simulink model "benign"  (R2017a)
settings: Solver=FixedStepDiscrete  StartTime=0.0  StopTime=100  FixedStep=1  RelTol=1e-3
model workspace (MAT data in the model file):
  MCOS : class17 (value not decoded)
undefined symbols (not defined in the file or in its folder): contractAfterSimulation, contractBeforeSimulation, saveValidatorParameters
undefined symbols (not defined in the file): ContractBlock, ContractGuaranteeBlock, ContractValidatorBlock
libraries: simulink x436, CoCoSimSpecification x31
(part 2 of 3)

== system benign/uas/autonomous_flight ==
  dest_reached : Inport  OutDataTypeStr=boolean
  payload_performed : Inport  Port=2  OutDataTypeStr=boolean
  mission1_waypoint_x : Inport  Port=3  OutDataTypeStr=int32
  mission1_waypoint_y : Inport  Port=4  OutDataTypeStr=int32
  mission1_payload : Inport  Port=5  OutDataTypeStr=int32
  mission1_status : Inport  Port=6  OutDataTypeStr=int32
  mission2_waypoint_x : Inport  Port=7  OutDataTypeStr=int32
  mission2_waypoint_y : Inport  Port=8  OutDataTypeStr=int32
  mission2_payload : Inport  Port=9  OutDataTypeStr=int32
  mission2_status : Inport  Port=10  OutDataTypeStr=int32
  mission3_waypoint_x : Inport  Port=11  OutDataTypeStr=int32
  mission3_waypoint_y : Inport  Port=12  OutDataTypeStr=int32
  mission3_payload : Inport  Port=13  OutDataTypeStr=int32
  mission3_status : Inport  Port=14  OutDataTypeStr=int32
  mstate : Inport  Port=15  OutDataTypeStr=int32
  payload : Subsystem
  upd_1_status : Subsystem
  upd_2_status : Subsystem
  upd_3_status : Subsystem
  waypoint_x : Subsystem
  waypoint_y : Subsystem
  upd_mission1_waypoint_x : Outport  OutDataTypeStr=int32
  upd_mission1_waypoint_y : Outport  Port=2  OutDataTypeStr=int32
  upd_mission1_payload : Outport  Port=3  OutDataTypeStr=int32
  upd_mission1_status : Outport  Port=4  OutDataTypeStr=int32
  upd_mission2_waypoint_x : Outport  Port=5  OutDataTypeStr=int32
  upd_mission2_waypoint_y : Outport  Port=6  OutDataTypeStr=int32
  upd_mission2_payload : Outport  Port=7  OutDataTypeStr=int32
  upd_mission2_status : Outport  Port=8  OutDataTypeStr=int32
  upd_mission3_waypoint_x : Outport  Port=9  OutDataTypeStr=int32
  upd_mission3_waypoint_y : Outport  Port=10  OutDataTypeStr=int32
  upd_mission3_payload : Outport  Port=11  OutDataTypeStr=int32
  upd_mission3_status : Outport  Port=12  OutDataTypeStr=int32
  waypointPos_x : Outport  Port=13  OutDataTypeStr=int32
  waypointPos_y : Outport  Port=14  OutDataTypeStr=int32
  payloadCMD : Outport  Port=15  OutDataTypeStr=int32
  wires:
  payload/1(payloadCMD) -> payloadCMD/1
  dest_reached/1 -> payload/1(dest_reached), upd_3_status/1(dest_reached), upd_2_status/1(dest_reached), upd_1_status/1(dest_reached), waypoint_y/1(dest_reached), waypoint_x/1(dest_reached)
  payload_performed/1 -> payload/2(payload_performed), upd_3_status/2(payload_performed), upd_2_status/2(payload_performed), upd_1_status/2(payload_performed), waypoint_y/2(payload_performed), waypoint_x/2(payload_performed)
  mission1_payload/1 -> payload/3(mission1_payload), upd_mission1_payload/1
  mission1_status/1 -> payload/4(mission1_status), upd_3_status/3(mission1_status), upd_2_status/3(mission1_status), upd_1_status/3(mission1_status), waypoint_y/3(mission1_status), waypoint_x/3(mission1_status)
  mission2_payload/1 -> payload/5(mission2_payload), upd_mission2_payload/1
  mission2_status/1 -> payload/6(mission2_status), upd_3_status/4(mission2_status), upd_2_status/4(mission2_status), upd_1_status/4(mission2_status), waypoint_y/4(mission2_status), waypoint_x/4(mission2_status)
  mission3_payload/1 -> payload/7(mission3_payload), upd_mission3_payload/1
  mission3_status/1 -> payload/8(mission3_status), upd_3_status/5(mission3_status), upd_2_status/5(mission3_status), upd_1_status/5(mission3_status), waypoint_y/5(mission3_status), waypoint_x/5(mission3_status)
  mstate/1 -> payload/9(mstate), upd_3_status/6(mstate), upd_2_status/6(mstate), upd_1_status/6(mstate), waypoint_y/6(mstate), waypoint_x/6(mstate)
  waypoint_x/1(waypointPos_x) -> waypointPos_x/1
  mission1_waypoint_x/1 -> upd_mission1_waypoint_x/1, waypoint_x/7(mission1_waypoint_x)
  mission2_waypoint_x/1 -> upd_mission2_waypoint_x/1, waypoint_x/8(mission2_waypoint_x)
  mission3_waypoint_x/1 -> upd_mission3_waypoint_x/1, waypoint_x/9(mission3_waypoint_x)
  mission1_waypoint_y/1 -> upd_mission1_waypoint_y/1, waypoint_y/7(mission1_waypoint_y)
  mission2_waypoint_y/1 -> upd_mission2_waypoint_y/1, waypoint_y/8(mission2_waypoint_y)
  mission3_waypoint_y/1 -> upd_mission3_waypoint_y/1, waypoint_y/9(mission3_waypoint_y)
  waypoint_y/1(waypointPos_y) -> waypointPos_y/1
  upd_1_status/1(upd_mission1_status) -> upd_mission1_status/1
  upd_2_status/1(upd_mission2_status) -> upd_mission2_status/1
  upd_3_status/1(upd_mission3_status) -> upd_mission3_status/1

== system benign/uas/battery_health_check ==
  battery_level : Inport  OutDataTypeStr=int32
  Constant : Constant  OutDataTypeStr=int32
  Constant1 : Constant  Value=0  OutDataTypeStr=int32
  Constant2 : Constant  Value=-1  OutDataTypeStr=int32
  Logical Operator : Logic  IconShape=distinctive  AllPortsSameDT=off  OutDataTypeStr=boolean
  Relational Operator : RelationalOperator  Operator=>  OutDataTypeStr=boolean  RndMeth=Simplest
  Relational Operator1 : RelationalOperator  Operator=<=  OutDataTypeStr=boolean  RndMeth=Simplest
  Relational Operator2 : RelationalOperator  OutDataTypeStr=boolean  RndMeth=Simplest
  Switch : Switch  Criteria=u2 > Threshold
  Switch1 : Switch  Criteria=u2 > Threshold
  first_level : Constant  Value=10  OutDataTypeStr=int32
  second_level : Constant  Value=5  OutDataTypeStr=int32
  ATE7 : Outport  OutDataTypeStr=int32
  wires:
  battery_level/1 -> Relational Operator2/1, Relational Operator1/1, Relational Operator/1
  first_level/1 -> Relational Operator1/2, Relational Operator/2
  Switch/1 -> ATE7/1
  Relational Operator/1 -> Switch/2
  Constant/1 -> Switch/1
  Switch1/1 -> Switch/3
  Relational Operator1/1 -> Logical Operator/1
  Relational Operator2/1 -> Logical Operator/2
  second_level/1 -> Relational Operator2/2
  Logical Operator/1 -> Switch1/2
  Constant1/1 -> Switch1/1
  Constant2/1 -> Switch1/3

== system benign/uas/channel_afl2act ==
  in_payloadCMD : Inport  OutDataTypeStr=int32
  out_payloadCMD : Outport  OutDataTypeStr=int32
  wires:
  in_payloadCMD/1 -> out_payloadCMD/1

== system benign/uas/channel_gps2pes ==
  currPos_x : Inport  OutDataTypeStr=int32
  currPos_y : Inport  Port=2  OutDataTypeStr=int32
  currDir : Inport  Port=3  OutDataTypeStr=int32
  gps2pes_GPS_pos_x : Outport  OutDataTypeStr=int32
  gps2pes_GPS_pos_y : Outport  Port=2  OutDataTypeStr=int32
  gps2pes_GPS_dir : Outport  Port=3  OutDataTypeStr=int32
  wires:
  currPos_x/1 -> gps2pes_GPS_pos_x/1
  currPos_y/1 -> gps2pes_GPS_pos_y/1
  currDir/1 -> gps2pes_GPS_dir/1

== system benign/uas/channel_poe2mix_a ==
  in_dir : Inport  OutDataTypeStr=int32
  out_dir : Outport  OutDataTypeStr=int32
  wires:
  in_dir/1 -> out_dir/1

== system benign/uas/channel_poe2mix_b ==
  in_movement : Inport  OutDataTypeStr=int32
  out_movement : Outport  OutDataTypeStr=int32
  wires:
  in_movement/1 -> out_movement/1

== system benign/uas/done logic ==
  mission1_status : Inport  OutDataTypeStr=int32
  mission2_status : Inport  Port=2  OutDataTypeStr=int32
  mission3_status : Inport  Port=3  OutDataTypeStr=int32
  Compare To Constant : simulink/Logic and Bit Operations/Compare To Constant  relop===  const=0  OutDataTypeStr=boolean
  Compare To Constant1 : simulink/Logic and Bit Operations/Compare To Constant  relop===  const=0  OutDataTypeStr=boolean
  Compare To Constant2 : simulink/Logic and Bit Operations/Compare To Constant  relop===  const=0  OutDataTypeStr=boolean
  Compare To Constant3 : simulink/Logic and Bit Operations/Compare To Constant  relop===  const=1  OutDataTypeStr=boolean
  Compare To Constant4 : simulink/Logic and Bit Operations/Compare To Constant  relop===  const=1  OutDataTypeStr=boolean
  Compare To Constant5 : simulink/Logic and Bit Operations/Compare To Constant  relop===  const=1  OutDataTypeStr=boolean
  Logical Operator : Logic  Inputs=3  IconShape=distinctive  AllPortsSameDT=off  OutDataTypeStr=boolean
  Logical Operator1 : Logic  Inputs=3  IconShape=distinctive  AllPortsSameDT=off  OutDataTypeStr=boolean
  Switch : Switch  Criteria=u2 > Threshold
  Switch1 : Switch  Criteria=u2 > Threshold
  false : Constant  Value=0  OutDataTypeStr=boolean
  true : Constant  OutDataTypeStr=boolean
  true1 : Constant  OutDataTypeStr=boolean
  done : Outport  OutDataTypeStr=boolean
  wires:
  mission1_status/1 -> Compare To Constant/1, Compare To Constant3/1
  true/1 -> Switch/1
  Switch/1 -> done/1
  Logical Operator/1 -> Switch/2
  Compare To Constant/1 -> Logical Operator/1
  Compare To Constant1/1 -> Logical Operator/2
  mission2_status/1 -> Compare To Constant4/1, Compare To Constant1/1
  mission3_status/1 -> Compare To Constant5/1, Compare To Constant2/1
  Compare To Constant2/1 -> Logical Operator/3
  Compare To Constant3/1 -> Logical Operator1/1
  Compare To Constant4/1 -> Logical Operator1/2
  Compare To Constant5/1 -> Logical Operator1/3
  Logical Operator1/1 -> Switch1/2
  true1/1 -> Switch1/1
  false/1 -> Switch1/3
  Switch1/1 -> Switch/3

== system benign/uas/mission_planner ==
  dummy : Inport  OutDataTypeStr=boolean
  c{,1,3,7} (4 alike) : Constant  OutDataTypeStr=int32
  c10 : Constant  Value=3  OutDataTypeStr=int32
  c11 : Constant  Value=3  OutDataTypeStr=int32
  c{2,4..5,8} (4 alike) : Constant  Value=2  OutDataTypeStr=int32
  c6 : Constant  Value=0  OutDataTypeStr=int32
  c9 : Constant  Value=3  OutDataTypeStr=int32
  m1_waypoint_x : Outport  OutDataTypeStr=int32
  m1_waypoint_y : Outport  Port=2  OutDataTypeStr=int32
  m1_payload : Outport  Port=3  OutDataTypeStr=int32
  m1_status : Outport  Port=4  OutDataTypeStr=int32
  m2_waypoint_x : Outport  Port=5  OutDataTypeStr=int32
  m2_waypoint_y : Outport  Port=6  OutDataTypeStr=int32
  m2_payload : Outport  Port=7  OutDataTypeStr=int32
  m2_status : Outport  Port=8  OutDataTypeStr=int32
  m3_waypoint_x : Outport  Port=9  OutDataTypeStr=int32
  m3_waypoint_y : Outport  Port=10  OutDataTypeStr=int32
  m3_payload : Outport  Port=11  OutDataTypeStr=int32
  m3_status : Outport  Port=12  OutDataTypeStr=int32
  wires:
  c/1 -> m1_waypoint_x/1
  c1/1 -> m2_waypoint_x/1
  c2/1 -> m3_waypoint_x/1
  c3/1 -> m1_waypoint_y/1
  c4/1 -> m2_waypoint_y/1
  c5/1 -> m3_waypoint_y/1
  c6/1 -> m1_payload/1
  c7/1 -> m2_payload/1
  c8/1 -> m3_payload/1
  c9/1 -> m1_status/1
  c11/1 -> m3_status/1
  c10/1 -> m2_status/1

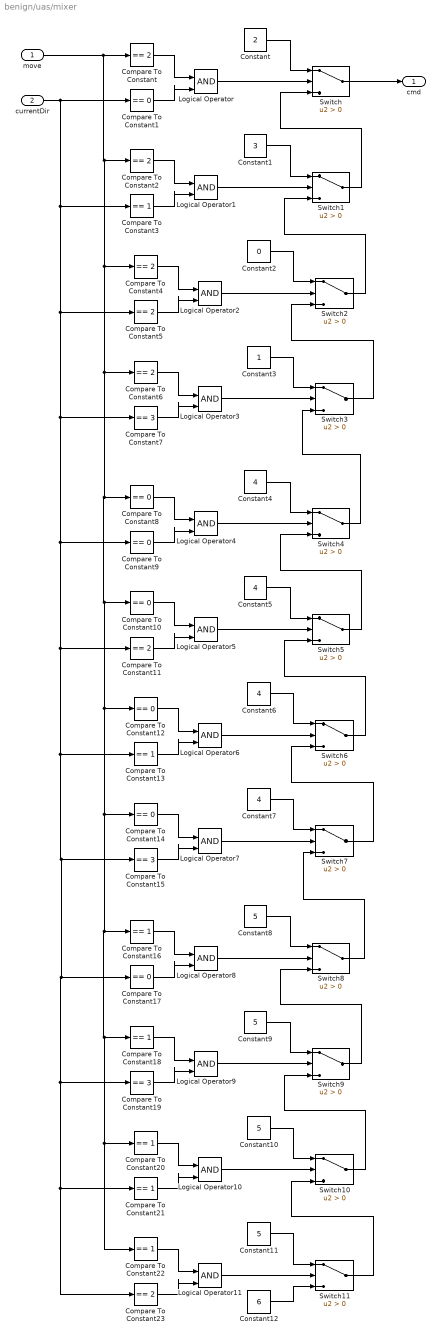
== system benign/uas/mixer ==
  move : Inport  OutDataTypeStr=int32
  currentDir : Inport  Port=2  OutDataTypeStr=int32
  Compare To Constant{,2,4..6,11,23} (7 alike) : simulink/Logic and Bit Operations/Compare To Constant  relop===  const=2  OutDataTypeStr=boolean
  Compare To Constant{1,8..10,12,14,17} (7 alike) : simulink/Logic and Bit Operations/Compare To Constant  relop===  const=0  OutDataTypeStr=boolean
  Compare To Constant{3,13,16,18,20..22} (7 alike) : simulink/Logic and Bit Operations/Compare To Constant  relop===  const=1  OutDataTypeStr=boolean
  Compare To Constant15 : simulink/Logic and Bit Operations/Compare To Constant  relop===  const=3  OutDataTypeStr=boolean
  Compare To Constant19 : simulink/Logic and Bit Operations/Compare To Constant  relop===  const=3  OutDataTypeStr=boolean
  Compare To Constant7 : simulink/Logic and Bit Operations/Compare To Constant  relop===  const=3  OutDataTypeStr=boolean
  Constant : Constant  Value=2  OutDataTypeStr=int32
  Constant1 : Constant  Value=3  OutDataTypeStr=int32
  Constant{8..11} (4 alike) : Constant  Value=5  OutDataTypeStr=int32
  Constant12 : Constant  Value=6  OutDataTypeStr=int32
  Constant2 : Constant  Value=0  OutDataTypeStr=int32
  Constant3 : Constant  OutDataTypeStr=int32
  Constant{4..7} (4 alike) : Constant  Value=4  OutDataTypeStr=int32
  Logical Operator{,1..11} (12 alike) : Logic  IconShape=distinctive  AllPortsSameDT=off  OutDataTypeStr=boolean
  Switch{,1..11} (12 alike) : Switch  Criteria=u2 > Threshold
  cmd : Outport  OutDataTypeStr=int32
  wires:
  Compare To Constant/1 -> Logical Operator/1
  Compare To Constant1/1 -> Logical Operator/2
  Logical Operator/1 -> Switch/2
  Switch/1 -> cmd/1
  Constant/1 -> Switch/1
  Logical Operator1/1 -> Switch1/2
  Compare To Constant2/1 -> Logical Operator1/1
  Switch1/1 -> Switch/3
  Compare To Constant3/1 -> Logical Operator1/2
  Constant1/1 -> Switch1/1
  Switch2/1 -> Switch1/3
  Compare To Constant4/1 -> Logical Operator2/1
  Constant2/1 -> Switch2/1
  Logical Operator2/1 -> Switch2/2
  Compare To Constant5/1 -> Logical Operator2/2
  Constant3/1 -> Switch3/1
  Switch3/1 -> Switch2/3
  Logical Operator3/1 -> Switch3/2
  Compare To Constant6/1 -> Logical Operator3/1
  Compare To Constant7/1 -> Logical Operator3/2
  Switch5/1 -> Switch4/3
  Logical Operator4/1 -> Switch4/2
  Logical Operator6/1 -> Switch6/2
  Constant6/1 -> Switch6/1
  Compare To Constant12/1 -> Logical Operator6/1
  Switch6/1 -> Switch5/3
  Switch7/1 -> Switch6/3
  Compare To Constant13/1 -> Logical Operator6/2
  Compare To Constant14/1 -> Logical Operator7/1
  Compare To Constant15/1 -> Logical Operator7/2
  Constant7/1 -> Switch7/1
  Compare To Constant8/1 -> Logical Operator4/1
  Logical Operator7/1 -> Switch7/2
  Switch4/1 -> Switch3/3
  Compare To Constant9/1 -> Logical Operator4/2
  Constant4/1 -> Switch4/1
  Constant5/1 -> Switch5/1
  Compare To Constant10/1 -> Logical Operator5/1
  Logical Operator5/1 -> Switch5/2
  Compare To Constant11/1 -> Logical Operator5/2
  Switch9/1 -> Switch8/3
  Logical Operator8/1 -> Switch8/2
  Logical Operator10/1 -> Switch10/2
  Constant10/1 -> Switch10/1
  Compare To Constant20/1 -> Logical Operator10/1
  Switch10/1 -> Switch9/3
  Switch11/1 -> Switch10/3
  Compare To Constant21/1 -> Logical Operator10/2
  Compare To Constant22/1 -> Logical Operator11/1
  Compare To Constant23/1 -> Logical Operator11/2
  Constant11/1 -> Switch11/1
  Compare To Constant16/1 -> Logical Operator8/1
  Logical Operator11/1 -> Switch11/2
  Switch8/1 -> Switch7/3
  Compare To Constant17/1 -> Logical Operator8/2
  currentDir/1 -> Compare To Constant5/1, Compare To Constant13/1, Compare To Constant21/1, Compare To Constant23/1, Compare To Constant19/1, Compare To Constant17/1, Compare To Constant15/1, Compare To Constant11/1, Compare To Constant9/1, Compare To Constant7/1, Compare To Constant3/1, Compare To Constant1/1
  Constant8/1 -> Switch8/1
  Constant9/1 -> Switch9/1
  Compare To Constant18/1 -> Logical Operator9/1
  move/1 -> Compare To Constant22/1, Compare To Constant20/1, Compare To Constant18/1, Compare To Constant16/1, Compare To Constant14/1, Compare To Constant12/1, Compare To Constant10/1, Compare To Constant8/1, Compare To Constant6/1, Compare To Constant4/1, Compare To Constant2/1, Compare To Constant/1
  Logical Operator9/1 -> Switch9/2
  Compare To Constant19/1 -> Logical Operator9/2
  Constant12/1 -> Switch11/3

== system benign/uas/navigator ==
  estimatedPos_x : Inport  OutDataTypeStr=int32
  estimatedPos_y : Inport  Port=2  OutDataTypeStr=int32
  waypointPos_x : Inport  Port=3  OutDataTypeStr=int32
  waypointPos_y : Inport  Port=4  OutDataTypeStr=int32
  Logical Operator : Logic  IconShape=distinctive  AllPortsSameDT=off  OutDataTypeStr=boolean
  Relational Operator : RelationalOperator  Operator===  OutDataTypeStr=boolean  RndMeth=Simplest
  Relational Operator1 : RelationalOperator  Operator===  OutDataTypeStr=boolean  RndMeth=Simplest
  dest_reached : Outport  OutDataTypeStr=boolean
  wires:
  estimatedPos_x/1 -> Relational Operator/1
  waypointPos_x/1 -> Relational Operator/2
  estimatedPos_y/1 -> Relational Operator1/1
  waypointPos_y/1 -> Relational Operator1/2
  Logical Operator/1 -> dest_reached/1
  Relational Operator/1 -> Logical Operator/1
  Relational Operator1/1 -> Logical Operator/2

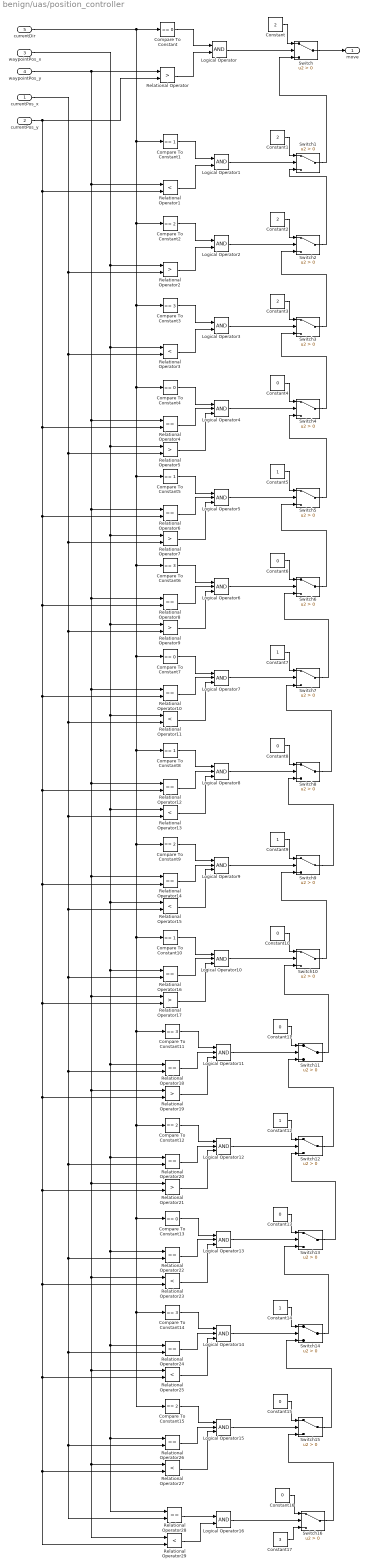
== system benign/uas/position_controller ==
  currentPos_x : Inport  OutDataTypeStr=int32
  currentPos_y : Inport  Port=2  OutDataTypeStr=int32
  waypointPos_x : Inport  Port=3  OutDataTypeStr=int32
  waypointPos_y : Inport  Port=4  OutDataTypeStr=int32
  currentDir : Inport  Port=5  OutDataTypeStr=int32
  Compare To Constant{,4,7,13} (4 alike) : simulink/Logic and Bit Operations/Compare To Constant  relop===  const=0  OutDataTypeStr=boolean
  Compare To Constant{1,5,8,10} (4 alike) : simulink/Logic and Bit Operations/Compare To Constant  relop===  const=1  OutDataTypeStr=boolean
  Compare To Constant{3,6,11,14} (4 alike) : simulink/Logic and Bit Operations/Compare To Constant  relop===  const=3  OutDataTypeStr=boolean
  Compare To Constant{2,9,12,15} (4 alike) : simulink/Logic and Bit Operations/Compare To Constant  relop===  const=2  OutDataTypeStr=boolean
  Constant{,1..3} (4 alike) : Constant  Value=2  OutDataTypeStr=int32
  Constant{4,6,8,10..11,13,15..16} (8 alike) : Constant  Value=0  OutDataTypeStr=int32
  Constant{5,7,9,12,14} (5 alike) : Constant  OutDataTypeStr=int32
  Constant17 : Constant  Value=3  OutDataTypeStr=int32
  Logical Operator{,1..3,16} (5 alike) : Logic  AllPortsSameDT=off  OutDataTypeStr=boolean
  Logical Operator{4..15} (12 alike) : Logic  Inputs=3  AllPortsSameDT=off  OutDataTypeStr=boolean
  Relational Operator{,2,5,7,9,17,19,21} (8 alike) : RelationalOperator  Operator=>  OutDataTypeStr=boolean  RndMeth=Simplest
  Relational Operator{1,3,11,13,15,23,25,27,29} (9 alike) : RelationalOperator  Operator=<  OutDataTypeStr=boolean  RndMeth=Simplest
  Relational Operator{4,6,8,10,12,14,16,18,20,22,24,26,28} (13 alike) : RelationalOperator  Operator===  OutDataTypeStr=boolean  RndMeth=Simplest
  Switch{,1..16} (17 alike) : Switch  Criteria=u2 > Threshold
  move : Outport  OutDataTypeStr=int32
  wires:
  Compare To Constant/1 -> Logical Operator/1
  Relational Operator/1 -> Logical Operator/2
  Logical Operator/1 -> Switch/2
  Switch/1 -> move/1
  Constant/1 -> Switch/1
  Constant1/1 -> Switch1/1
  Switch1/1 -> Switch/3
  Relational Operator1/1 -> Logical Operator1/2
  Logical Operator1/1 -> Switch1/2
  Compare To Constant1/1 -> Logical Operator1/1
  Switch2/1 -> Switch1/3
  Logical Operator2/1 -> Switch2/2
  Compare To Constant2/1 -> Logical Operator2/1
  Constant2/1 -> Switch2/1
  Relational Operator2/1 -> Logical Operator2/2
  Constant3/1 -> Switch3/1
  Compare To Constant3/1 -> Logical Operator3/1
  Relational Operator3/1 -> Logical Operator3/2
  Logical Operator3/1 -> Switch3/2
  Switch3/1 -> Switch2/3
  Relational Operator4/1 -> Logical Operator4/2
  Compare To Constant4/1 -> Logical Operator4/1
  Constant4/1 -> Switch4/1
  Logical Operator4/1 -> Switch4/2
  Switch4/1 -> Switch3/3
  Relational Operator5/1 -> Logical Operator4/3
  Constant5/1 -> Switch5/1
  Compare To Constant5/1 -> Logical Operator5/1
  Logical Operator5/1 -> Switch5/2
  Relational Operator7/1 -> Logical Operator5/3
  Relational Operator6/1 -> Logical Operator5/2
  Switch5/1 -> Switch4/3
  Switch6/1 -> Switch5/3
  Relational Operator8/1 -> Logical Operator6/2
  Constant6/1 -> Switch6/1
  Relational Operator9/1 -> Logical Operator6/3
  Compare To Constant6/1 -> Logical Operator6/1
  Logical Operator6/1 -> Switch6/2
  Logical Operator7/1 -> Switch7/2
  Compare To Constant7/1 -> Logical Operator7/1
  Relational Operator11/1 -> Logical Operator7/3
  Constant7/1 -> Switch7/1
  Relational Operator10/1 -> Logical Operator7/2
  Switch7/1 -> Switch6/3
  Compare To Constant8/1 -> Logical Operator8/1
  Logical Operator8/1 -> Switch8/2
  Relational Operator12/1 -> Logical Operator8/2
  Switch8/1 -> Switch7/3
  Constant8/1 -> Switch8/1
  Relational Operator13/1 -> Logical Operator8/3
  Switch9/1 -> Switch8/3
  Constant9/1 -> Switch9/1
  Relational Operator14/1 -> Logical Operator9/2
  Compare To Constant9/1 -> Logical Operator9/1
  Logical Operator9/1 -> Switch9/2
  Relational Operator15/1 -> Logical Operator9/3
  Relational Operator17/1 -> Logical Operator10/3
  Compare To Constant10/1 -> Logical Operator10/1
  Constant10/1 -> Switch10/1
  Logical Operator10/1 -> Switch10/2
  Switch10/1 -> Switch9/3
  Relational Operator16/1 -> Logical Operator10/2
  Logical Operator11/1 -> Switch11/2
  Constant11/1 -> Switch11/1
  Compare To Constant11/1 -> Logical Operator11/1
  Relational Operator19/1 -> Logical Operator11/3
  Switch11/1 -> Switch10/3
  Relational Operator18/1 -> Logical Operator11/2
  Switch12/1 -> Switch11/3
  Relational Operator20/1 -> Logical Operator12/2
  Compare To Constant12/1 -> Logical Operator12/1
  Constant12/1 -> Switch12/1
  Relational Operator21/1 -> Logical Operator12/3
  Logical Operator12/1 -> Switch12/2
  Relational Operator23/1 -> Logical Operator13/3
  Compare To Constant13/1 -> Logical Operator13/1
  Relational Operator22/1 -> Logical Operator13/2
  Constant13/1 -> Switch13/1
  Logical Operator13/1 -> Switch13/2
  Switch13/1 -> Switch12/3
  Relational Operator24/1 -> Logical Operator14/2
  Switch14/1 -> Switch13/3
  Logical Operator14/1 -> Switch14/2
  Constant14/1 -> Switch14/1
  Compare To Constant14/1 -> Logical Operator14/1
  Relational Operator25/1 -> Logical Operator14/3
  Relational Operator27/1 -> Logical Operator15/3
  Relational Operator26/1 -> Logical Operator15/2
  Logical Operator15/1 -> Switch15/2
  Constant15/1 -> Switch15/1
  Compare To Constant15/1 -> Logical Operator15/1
  Switch15/1 -> Switch14/3
  currentDir/1 -> Compare To Constant5/1, Compare To Constant6/1, Compare To Constant7/1, Compare To Constant8/1, Compare To Constant9/1, Compare To Constant10/1, Compare To Constant12/1, Compare To Constant13/1, Compare To Constant14/1, Compare To Constant15/1, Compare To Constant11/1, Compare To Constant4/1, Compare To Constant3/1, Compare To Constant2/1, Compare To Constant1/1, Compare To Constant/1
  waypointPos_x/1 -> Relational Operator5/1, Relational Operator7/1, Relational Operator9/1, Relational Operator11/1, Relational Operator13/1, Relational Operator15/1, Relational Operator16/1, Relational Operator20/1, Relational Operator22/1, Relational Operator24/1, Relational Operator26/1, Relational Operator28/1, Relational Operator18/1, Relational Operator3/1, Relational Operator2/1
  currentPos_y/1 -> Relational Operator6/2, Relational Operator8/2, Relational Operator10/2, Relational Operator12/2, Relational Operator14/2, Relational Operator17/2, Relational Operator21/2, Relational Operator23/2, Relational Operator25/2, Relational Operator27/2, Relational Operator29/2, Relational Operator19/2, Relational Operator4/2, Relational Operator1/2, Relational Operator/2
  Constant16/1 -> Switch16/1
  Relational Operator28/1 -> Logical Operator16/1
  Logical Operator16/1 -> Switch16/2
  waypointPos_y/1 -> Relational Operator/1, Relational Operator4/1, Relational Operator6/1, Relational Operator8/1, Relational Operator10/1, Relational Operator12/1, Relational Operator14/1, Relational Operator17/1, Relational Operator21/1, Relational Operator23/1, Relational Operator25/1, Relational Operator27/1, Relational Operator29/1, Relational Operator19/1, Relational Operator1/1
  Switch16/1 -> Switch15/3
  currentPos_x/1 -> Relational Operator7/2, Relational Operator9/2, Relational Operator11/2, Relational Operator13/2, Relational Operator15/2, Relational Operator16/2, Relational Operator20/2, Relational Operator22/2, Relational Operator24/2, Relational Operator26/2, Relational Operator28/2, Relational Operator18/2, Relational Operator5/2, Relational Operator3/2, Relational Operator2/2
  Relational Operator29/1 -> Logical Operator16/2
  Constant17/1 -> Switch16/3

== system benign/uas/position_estimator ==
  gps2pes_GPS_pos_x : Inport  OutDataTypeStr=int32
  gps2pes_GPS_pos_y : Inport  Port=2  OutDataTypeStr=int32
  gps2pes_GPS_dir : Inport  Port=3  OutDataTypeStr=int32
  currPos_x : Inport  Port=4  OutDataTypeStr=int32
  currPos_y : Inport  Port=5  OutDataTypeStr=int32
  currDir : Inport  Port=6  OutDataTypeStr=int32
  estimatedPos_x : Outport  OutDataTypeStr=int32
  estimatedPos_y : Outport  Port=2  OutDataTypeStr=int32
  estimatedDir : Outport  Port=3  OutDataTypeStr=int32
  wires:
  gps2pes_GPS_pos_x/1 -> estimatedPos_x/1
  gps2pes_GPS_pos_y/1 -> estimatedPos_y/1
  gps2pes_GPS_dir/1 -> estimatedDir/1

== system benign/uas/state_machine ==
  ATE6 : Inport
  ATE7 : Inport  Port=2
  six : Constant  Value=6  OutDataTypeStr=int32
  mstate : Outport  OutDataTypeStr=int32
  wires:
  six/1 -> mstate/1

== system benign/uas/yaw2dir ==
  yaw : Inport  OutDataTypeStr=int32
  Switch : Switch  Criteria=u2 > Threshold
  Switch1 : Switch  Criteria=u2 > Threshold
  Switch2 : Switch  Criteria=u2 > Threshold
  c0 : Constant  Value=0  OutDataTypeStr=int32
  c1 : Constant  OutDataTypeStr=int32
  c2 : Constant  Value=2  OutDataTypeStr=int32
  c3 : Constant  Value=3  OutDataTypeStr=int32
  yaw == 0 : simulink/Logic and Bit Operations/Compare To Constant  relop===  const=0  OutDataTypeStr=boolean
  yaw == 1 : simulink/Logic and Bit Operations/Compare To Constant  relop===  const=1  OutDataTypeStr=boolean
  yaw == 2 : simulink/Logic and Bit Operations/Compare To Constant  relop===  const=2  OutDataTypeStr=boolean
  dir : Outport  OutDataTypeStr=int32
  wires:
  yaw/1 -> yaw == 2/1, yaw == 1/1, yaw == 0/1
  yaw == 0/1 -> Switch/2
  c0/1 -> Switch/1
  Switch/1 -> dir/1
  yaw == 1/1 -> Switch1/2
  c2/1 -> Switch1/1
  Switch1/1 -> Switch/3
  yaw == 2/1 -> Switch2/2
  c1/1 -> Switch2/1
  c3/1 -> Switch2/3
  Switch2/1 -> Switch1/3

== system benign/uas/RC_receiver_health_check/duration ==
  p : Inport  OutDataTypeStr=boolean
  Add : Sum
  Constant : Constant  OutDataTypeStr=int32
  Constant1 : Constant  Value=0  OutDataTypeStr=int32
  Constant2 : Constant  Value=0  OutDataTypeStr=int32
  Constant3 : Constant  OutDataTypeStr=int32
  Logical Operator : Logic  Operator=NOT  IconShape=distinctive  AllPortsSameDT=off  OutDataTypeStr=boolean
  Switch : Switch  Criteria=u2 > Threshold
  Switch1 : Switch  Criteria=u2 > Threshold
  Unit Delay : UnitDelay  SampleTime=-1
  arrow1 : CoCoSimSpecification/arrow  LustreOperatorBlock=ArrowOperator
      settings: SourceProductName=CoCoSim Specification
  r : Outport  OutDataTypeStr=int32
  wires:
  Switch/1 -> arrow1/1
  arrow1/1 -> Unit Delay/1, r/1
  p/1 -> Logical Operator/1
  Logical Operator/1 -> Switch1/2, Switch/2
  Switch1/1 -> arrow1/2
  Constant/1 -> Switch/1
  Constant1/1 -> Switch/3
  Constant2/1 -> Switch1/3
  Constant3/1 -> Add/1
  Unit Delay/1 -> Add/2
  Add/1 -> Switch1/1

== system benign/uas/actuator/Subsystem ==
  cmd : Inport  OutDataTypeStr=int32
  Compare To Constant : simulink/Logic and Bit Operations/Compare To Constant  relop===  const=2  OutDataTypeStr=boolean
  Compare To Constant1 : simulink/Logic and Bit Operations/Compare To Constant  relop===  const=0  OutDataTypeStr=boolean
  Compare To Constant2 : simulink/Logic and Bit Operations/Compare To Constant  relop===  const=3  OutDataTypeStr=boolean
  Compare To Constant3 : simulink/Logic and Bit Operations/Compare To Constant  relop===  const=1  OutDataTypeStr=boolean
  Compare To Constant4 : simulink/Logic and Bit Operations/Compare To Constant  relop===  const=6  OutDataTypeStr=boolean
  Switch{,1..4} (5 alike) : Switch  Criteria=u2 > Threshold
  false : Constant  OutDataTypeStr=boolean
  true{,1..4} (5 alike) : Constant  OutDataTypeStr=boolean
  battery4pos_consumed : Outport
  wires:
  Switch/1 -> battery4pos_consumed/1
  true/1 -> Switch/1
  Compare To Constant/1 -> Switch/2
  Switch1/1 -> Switch/3
  Switch2/1 -> Switch1/3
  Switch3/1 -> Switch2/3
  true1/1 -> Switch1/1
  Compare To Constant1/1 -> Switch1/2
  true2/1 -> Switch2/1
  Compare To Constant2/1 -> Switch2/2
  true3/1 -> Switch3/1
  Compare To Constant3/1 -> Switch3/2
  Switch4/1 -> Switch3/3
  Compare To Constant4/1 -> Switch4/2
  true4/1 -> Switch4/1
  cmd/1 -> Compare To Constant2/1, Compare To Constant4/1, Compare To Constant3/1, Compare To Constant1/1, Compare To Constant/1
  false/1 -> Switch4/3

== system benign/uas/actuator/Subsystem1 ==
  cmd : Inport  OutDataTypeStr=int32
  currentPos_x : Inport  Port=2  OutDataTypeStr=int32
  Add : Sum
  Add1 : Sum
  Compare To Constant : simulink/Logic and Bit Operations/Compare To Constant  relop===  const=2  OutDataTypeStr=boolean
  Compare To Constant1 : simulink/Logic and Bit Operations/Compare To Constant  relop===  const=0  OutDataTypeStr=boolean
  Compare To Constant2 : simulink/Logic and Bit Operations/Compare To Constant  relop===  const=3  OutDataTypeStr=boolean
  Compare To Constant3 : simulink/Logic and Bit Operations/Compare To Constant  relop===  const=1  OutDataTypeStr=boolean
  Compare To Constant4 : simulink/Logic and Bit Operations/Compare To Constant  relop===  const=6  OutDataTypeStr=boolean
  Constant : Constant  OutDataTypeStr=int32
  Constant1 : Constant  Value=-1  OutDataTypeStr=int32
  Switch{,1..4} (5 alike) : Switch  Criteria=u2 > Threshold
  nextPos_x : Outport
  wires:
  cmd/1 -> Compare To Constant/1, Compare To Constant1/1, Compare To Constant3/1, Compare To Constant4/1, Compare To Constant2/1
  Compare To Constant4/1 -> Switch4/2
  Switch4/1 -> Switch3/3
  Compare To Constant3/1 -> Switch3/2
  Compare To Constant2/1 -> Switch2/2
  Compare To Constant1/1 -> Switch1/2
  Switch3/1 -> Switch2/3
  Switch2/1 -> Switch1/3
  Switch1/1 -> Switch/3
  Compare To Constant/1 -> Switch/2
  Switch/1 -> nextPos_x/1
  Constant/1 -> Add/2
  Add/1 -> Switch1/1
  Add1/1 -> Switch3/1
  Constant1/1 -> Add1/2
  currentPos_x/1 -> Switch4/3, Switch4/1, Add1/1, Switch2/1, Add/1, Switch/1

== system benign/uas/actuator/Subsystem2 ==
  cmd : Inport  OutDataTypeStr=int32
  currentPos_y : Inport  Port=2  OutDataTypeStr=int32
  Add2 : Sum
  Add3 : Sum
  Compare To Constant : simulink/Logic and Bit Operations/Compare To Constant  relop===  const=2  OutDataTypeStr=boolean
  Compare To Constant1 : simulink/Logic and Bit Operations/Compare To Constant  relop===  const=0  OutDataTypeStr=boolean
  Compare To Constant2 : simulink/Logic and Bit Operations/Compare To Constant  relop===  const=3  OutDataTypeStr=boolean
  Compare To Constant3 : simulink/Logic and Bit Operations/Compare To Constant  relop===  const=1  OutDataTypeStr=boolean
  Compare To Constant4 : simulink/Logic and Bit Operations/Compare To Constant  relop===  const=6  OutDataTypeStr=boolean
  Constant2 : Constant  OutDataTypeStr=int32
  Constant3 : Constant  Value=-1  OutDataTypeStr=int32
  Switch{,1..4} (5 alike) : Switch  Criteria=u2 > Threshold
  nextPos_y : Outport
  wires:
  currentPos_y/1 -> Add2/1, Switch1/1, Add3/1, Switch4/1, Switch4/3, Switch3/1
  Switch/1 -> nextPos_y/1
  Compare To Constant/1 -> Switch/2
  Switch1/1 -> Switch/3
  Switch2/1 -> Switch1/3
  Switch3/1 -> Switch2/3
  Compare To Constant1/1 -> Switch1/2
  Compare To Constant2/1 -> Switch2/2
  Compare To Constant3/1 -> Switch3/2
  Switch4/1 -> Switch3/3
  Compare To Constant4/1 -> Switch4/2
  cmd/1 -> Compare To Constant2/1, Compare To Constant4/1, Compare To Constant3/1, Compare To Constant1/1, Compare To Constant/1
  Constant2/1 -> Add2/2
  Add2/1 -> Switch/1
  Constant3/1 -> Add3/2
  Add3/1 -> Switch2/1

== system benign/uas/actuator/choose_battery_consumption ==
  i : Inport  OutDataTypeStr=int32
  one : Constant  OutDataTypeStr=int32
  o : Outport  OutDataTypeStr=int32
  wires:
  one/1 -> o/1

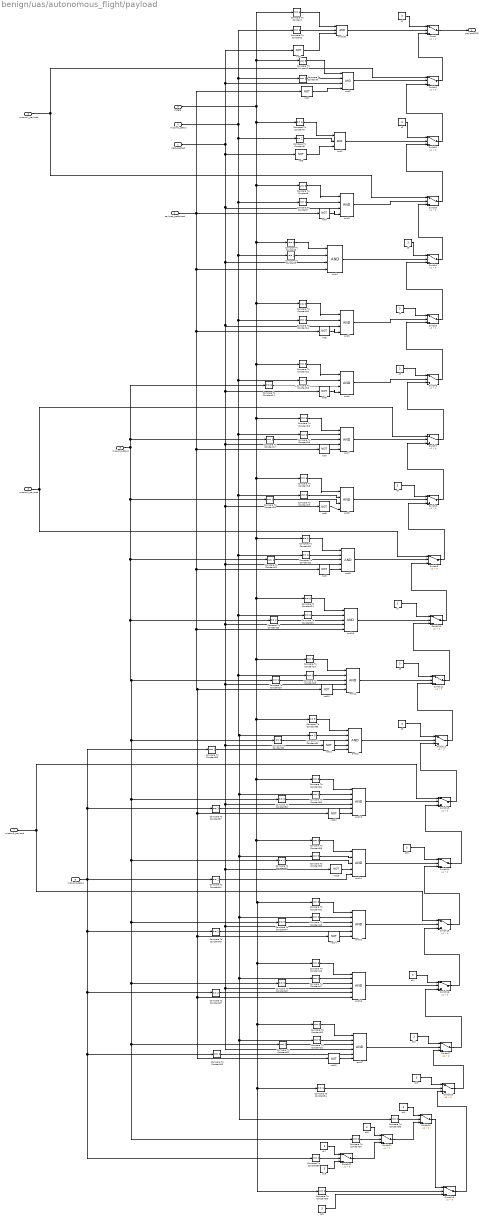
== system benign/uas/autonomous_flight/payload ==
  dest_reached : Inport  OutDataTypeStr=boolean
  payload_performed : Inport  Port=2  OutDataTypeStr=boolean
  mission1_payload : Inport  Port=3  OutDataTypeStr=int32
  mission1_status : Inport  Port=4  OutDataTypeStr=int32
  mission2_payload : Inport  Port=5  OutDataTypeStr=int32
  mission2_status : Inport  Port=6  OutDataTypeStr=int32
  mission3_payload : Inport  Port=7  OutDataTypeStr=int32
  mission3_status : Inport  Port=8  OutDataTypeStr=int32
  mstate : Inport  Port=9  OutDataTypeStr=int32
  Compare To Constant{,2,4,6,8,10,12,15,18,21,24,27,30,34,38,42,46,50} (18 alike) : simulink/Logic and Bit Operations/Compare To Constant  relop===  const=6  OutDataTypeStr=boolean
  Compare To Constant{1,3,14,17,33,37,54} (7 alike) : simulink/Logic and Bit Operations/Compare To Constant  relop===  const=3  OutDataTypeStr=boolean
  Compare To Constant{5,7,9,11,20,23,26,29,41,45,49,53,56..58} (15 alike) : simulink/Logic and Bit Operations/Compare To Constant  relop===  const=2  OutDataTypeStr=boolean
  Compare To Constant{13,16,19,22,25,28,31..32,35..36,39..40,43..44,47..48,51..52} (18 alike) : simulink/Logic and Bit Operations/Compare To Constant  relop===  const=0  OutDataTypeStr=boolean
  Compare To Constant55 : simulink/Logic and Bit Operations/Compare To Constant  relop===  const=4  OutDataTypeStr=boolean
  Switch{,1..22} (23 alike) : Switch  Criteria=u2 > Threshold
  and1 : Logic  Inputs=3  IconShape=distinctive  AllPortsSameDT=off  OutDataTypeStr=boolean
  and{7,9..12,14} (6 alike) : Logic  Inputs=5  IconShape=distinctive  AllPortsSameDT=off  OutDataTypeStr=boolean
  and101 : Logic  Inputs=3  IconShape=distinctive  AllPortsSameDT=off  OutDataTypeStr=boolean
  and{13,15..17} (4 alike) : Logic  Inputs=6  IconShape=distinctive  AllPortsSameDT=off  OutDataTypeStr=boolean
  and{2..6,8} (6 alike) : Logic  Inputs=4  IconShape=distinctive  AllPortsSameDT=off  OutDataTypeStr=boolean
  c{1..18} (18 alike) : Constant  Value=3  OutDataTypeStr=int32
  not{1..15} (15 alike) : Logic  Operator=NOT  Inputs=3  IconShape=distinctive  AllPortsSameDT=off  OutDataTypeStr=boolean
  payloadCMD : Outport  OutDataTypeStr=int32
  wires:
  Switch/1 -> payloadCMD/1
  c1/1 -> Switch/1
  and101/1 -> Switch/2
  Compare To Constant/1 -> and101/1
  Compare To Constant1/1 -> and101/2
  not1/1 -> and101/3
  Compare To Constant3/1 -> and2/2
  Compare To Constant2/1 -> and2/1
  Switch1/1 -> Switch/3
  and2/1 -> Switch1/2
  not2/1 -> and2/4
  Switch2/1 -> Switch1/3
  Compare To Constant4/1 -> and1/1
  c2/1 -> Switch2/1
  Compare To Constant5/1 -> and1/2
  and1/1 -> Switch2/2
  not3/1 -> and1/3
  and3/1 -> Switch3/2
  Compare To Constant7/1 -> and3/2
  Switch3/1 -> Switch2/3
  Compare To Constant6/1 -> and3/1
  not4/1 -> and3/4
  Compare To Constant8/1 -> and4/1
  and4/1 -> Switch4/2
  Compare To Constant9/1 -> and4/2
  Switch4/1 -> Switch3/3
  c3/1 -> Switch4/1
  Compare To Constant10/1 -> and5/1
  Compare To Constant11/1 -> and5/2
  and5/1 -> Switch5/2
  mission1_payload/1 -> Switch3/1, Switch1/1
  not5/1 -> and5/4
  Switch5/1 -> Switch4/3
  c4/1 -> Switch5/1
  Compare To Constant13/1 -> and6/2
  Compare To Constant12/1 -> and6/1
  not6/1 -> and6/4
  Switch6/1 -> Switch5/3
  c5/1 -> Switch6/1
  and6/1 -> Switch6/2
  Compare To Constant14/1 -> and6/3
  Compare To Constant17/1 -> and7/3
  and7/1 -> Switch7/2
  Compare To Constant16/1 -> and7/2
  Compare To Constant15/1 -> and7/1
  Switch7/1 -> Switch6/3
  not7/1 -> and7/5
  mission2_payload/1 -> Switch9/1, Switch7/1
  Compare To Constant18/1 -> and8/1
  Compare To Constant20/1 -> and8/3
  and8/1 -> Switch8/2
  Switch8/1 -> Switch7/3
  Compare To Constant19/1 -> and8/2
  not8/1 -> and8/4
  c6/1 -> Switch8/1
  Switch9/1 -> Switch8/3
  Compare To Constant21/1 -> and9/1
  Compare To Constant23/1 -> and9/3
  and9/1 -> Switch9/2
  Compare To Constant22/1 -> and9/2
  not9/1 -> and9/5
  Switch10/1 -> Switch9/3
  and10/1 -> Switch10/2
  Compare To Constant24/1 -> and10/1
  Compare To Constant26/1 -> and10/3
  Compare To Constant25/1 -> and10/2
  c7/1 -> Switch10/1
  c8/1 -> Switch11/1
  Switch11/1 -> Switch10/3
  Compare To Constant29/1 -> and11/3
  and11/1 -> Switch11/2
  Compare To Constant28/1 -> and11/2
  Compare To Constant27/1 -> and11/1
  not10/1 -> and11/5
  c9/1 -> Switch12/1
  Compare To Constant30/1 -> and12/1
  Switch12/1 -> Switch11/3
  Compare To Constant31/1 -> and12/2
  and12/1 -> Switch12/2
  Compare To Constant32/1 -> and12/3
  not11/1 -> and12/4
  Compare To Constant33/1 -> and12/5
  Switch13/1 -> Switch12/3
  Compare To Constant37/1 -> and13/5
  and13/1 -> Switch13/2
  Compare To Constant34/1 -> and13/1
  Compare To Constant35/1 -> and13/2
  Compare To Constant36/1 -> and13/3
  not12/1 -> and13/6
  Compare To Constant40/1 -> and14/3
  Compare To Constant39/1 -> and14/2
  Compare To Constant38/1 -> and14/1
  Compare To Constant41/1 -> and14/5
  Switch14/1 -> Switch13/3
  and14/1 -> Switch14/2
  c10/1 -> Switch14/1
  not13/1 -> and14/4
  and15/1 -> Switch15/2
  Compare To Constant45/1 -> and15/5
  Compare To Constant44/1 -> and15/3
  Switch15/1 -> Switch14/3
  not14/1 -> and15/6
  Compare To Constant42/1 -> and15/1
  Compare To Constant43/1 -> and15/2
  mission3_payload/1 -> Switch13/1, Switch15/1
  Switch16/1 -> Switch15/3
  Compare To Constant46/1 -> and16/1
  and16/1 -> Switch16/2
  Compare To Constant48/1 -> and16/3
  Compare To Constant47/1 -> and16/2
  Compare To Constant49/1 -> and16/5
  c11/1 -> Switch16/1
  and17/1 -> Switch17/2
  payload_performed/1 -> not2/1, not15/1, and16/6, not14/1, not12/1, not10/1, and10/5, not9/1, not7/1, not5/1, and4/4, not4/1
  c12/1 -> Switch17/1
  Compare To Constant51/1 -> and17/2
  mission2_status/1 -> Compare To Constant14/1, Compare To Constant17/1, Compare To Constant57/1, Compare To Constant52/1, Compare To Constant48/1, Compare To Constant44/1, Compare To Constant40/1, Compare To Constant36/1, Compare To Constant32/1, Compare To Constant29/1, Compare To Constant26/1, Compare To Constant23/1, Compare To Constant20/1
  dest_reached/1 -> and2/3, not1/1, and9/4, and16/4, and17/4, and15/4, not13/1, and13/4, not11/1, and11/4, and10/4, not8/1, and7/4, not6/1, and5/3, and4/3, and3/3, not3/1
  Compare To Constant53/1 -> and17/5
  Compare To Constant50/1 -> and17/1
  mission1_status/1 -> Compare To Constant7/1, Compare To Constant56/1, Compare To Constant51/1, Compare To Constant47/1, Compare To Constant43/1, Compare To Constant39/1, Compare To Constant35/1, Compare To Constant31/1, Compare To Constant28/1, Compare To Constant25/1, Compare To Constant22/1, Compare To Constant19/1, Compare To Constant16/1, Compare To Constant13/1, Compare To Constant11/1, Compare To Constant9/1, Compare To Constant5/1, Compare To Constant3/1, Compare To Constant1/1
  Compare To Constant52/1 -> and17/3
  Switch17/1 -> Switch16/3
  not15/1 -> and17/6
  Switch18/1 -> Switch17/3
  Compare To Constant54/1 -> Switch18/2
  c13/1 -> Switch18/1
  Switch19/1 -> Switch18/3
  mstate/1 -> Compare To Constant6/1, Compare To Constant12/1, Compare To Constant27/1, Compare To Constant55/1, Compare To Constant54/1, Compare To Constant50/1, Compare To Constant46/1, Compare To Constant42/1, Compare To Constant38/1, Compare To Constant34/1, Compare To Constant30/1, Compare To Constant24/1, Compare To Constant21/1, Compare To Constant18/1, Compare To Constant15/1, Compare To Constant10/1, Compare To Constant8/1, Compare To Constant4/1, Compare To Constant2/1, Compare To Constant/1
  c15/1 -> Switch19/3
  Compare To Constant55/1 -> Switch19/2
  Compare To Constant56/1 -> Switch20/2
  c14/1 -> Switch20/1
  Switch20/1 -> Switch19/1
  c16/1 -> Switch21/1
  Compare To Constant57/1 -> Switch21/2
  Switch21/1 -> Switch20/3
  Compare To Constant58/1 -> Switch22/2
  Switch22/1 -> Switch21/3
  c17/1 -> Switch22/1
  mission3_status/1 -> Compare To Constant33/1, Compare To Constant37/1, Compare To Constant49/1, Compare To Constant58/1, Compare To Constant53/1, Compare To Constant45/1, Compare To Constant41/1
  c18/1 -> Switch22/3

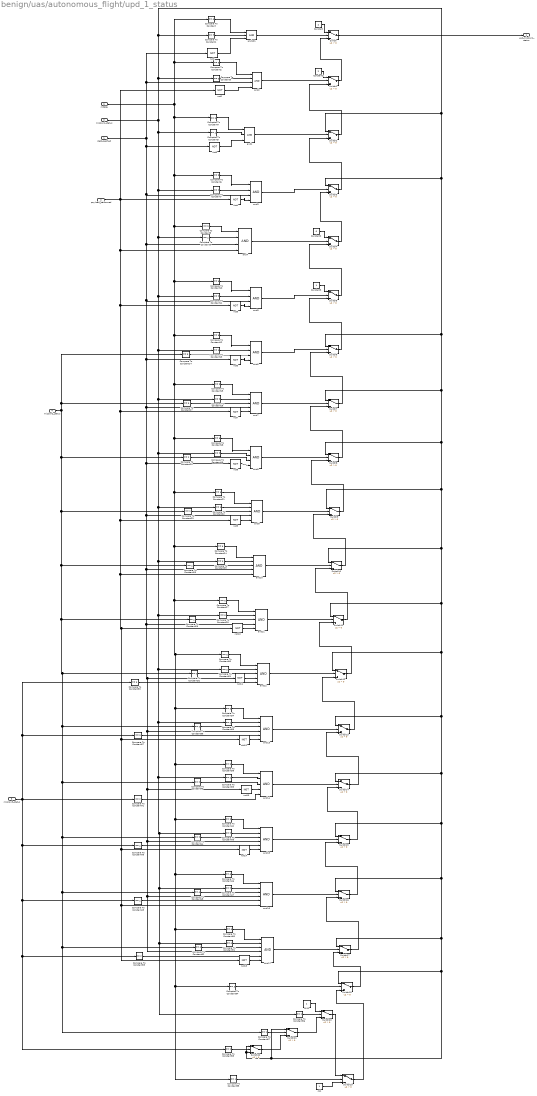
== system benign/uas/autonomous_flight/upd_1_status ==
  dest_reached : Inport  OutDataTypeStr=boolean
  payload_performed : Inport  Port=2  OutDataTypeStr=boolean
  mission1_status : Inport  Port=3  OutDataTypeStr=int32
  mission2_status : Inport  Port=4  OutDataTypeStr=int32
  mission3_status : Inport  Port=5  OutDataTypeStr=int32
  mstate : Inport  Port=6  OutDataTypeStr=int32
  Compare To Constant{,2,4,6,8,10,12,15,18,21,24,27,30,34,38,42,46,50} (18 alike) : simulink/Logic and Bit Operations/Compare To Constant  relop===  const=6  OutDataTypeStr=boolean
  Compare To Constant{1,3,14,17,33,37,54} (7 alike) : simulink/Logic and Bit Operations/Compare To Constant  relop===  const=3  OutDataTypeStr=boolean
  Compare To Constant{5,7,9,11,20,23,26,29,41,45,49,53,56..58} (15 alike) : simulink/Logic and Bit Operations/Compare To Constant  relop===  const=2  OutDataTypeStr=boolean
  Compare To Constant{13,16,19,22,25,28,31..32,35..36,39..40,43..44,47..48,51..52} (18 alike) : simulink/Logic and Bit Operations/Compare To Constant  relop===  const=0  OutDataTypeStr=boolean
  Compare To Constant55 : simulink/Logic and Bit Operations/Compare To Constant  relop===  const=4  OutDataTypeStr=boolean
  Constant : Constant  Value=2  OutDataTypeStr=int32
  Constant1 : Constant  Value=2  OutDataTypeStr=int32
  Constant2 : Constant  Value=0  OutDataTypeStr=int32
  Constant3 : Constant  OutDataTypeStr=int32
  Switch{,1..22} (23 alike) : Switch  Criteria=u2 > Threshold
  and1 : Logic  Inputs=3  IconShape=distinctive  AllPortsSameDT=off  OutDataTypeStr=boolean
  and{7,9..12,14} (6 alike) : Logic  Inputs=5  IconShape=distinctive  AllPortsSameDT=off  OutDataTypeStr=boolean
  and101 : Logic  Inputs=3  IconShape=distinctive  AllPortsSameDT=off  OutDataTypeStr=boolean
  and{13,15..17} (4 alike) : Logic  Inputs=6  IconShape=distinctive  AllPortsSameDT=off  OutDataTypeStr=boolean
  and{2..6,8} (6 alike) : Logic  Inputs=4  IconShape=distinctive  AllPortsSameDT=off  OutDataTypeStr=boolean
  c11 : Constant  OutDataTypeStr=int32
  c111 : Constant  OutDataTypeStr=int32
  not{1..15} (15 alike) : Logic  Operator=NOT  Inputs=3  IconShape=distinctive  AllPortsSameDT=off  OutDataTypeStr=boolean
  upd_mission1_status : Outport  OutDataTypeStr=int32
  wires:
  payload_performed/1 -> not4/1, and4/4, not5/1, not7/1, not9/1, and10/5, not10/1, not12/1, not14/1, and16/6, not15/1, not2/1
  mission3_status/1 -> Compare To Constant41/1, Compare To Constant45/1, Compare To Constant53/1, Compare To Constant58/1, Compare To Constant49/1, Compare To Constant37/1, Compare To Constant33/1
  Switch22/1 -> Switch21/3
  Compare To Constant58/1 -> Switch22/2
  Switch21/1 -> Switch20/3
  Compare To Constant57/1 -> Switch21/2
  Switch20/1 -> Switch19/1
  c111/1 -> Switch20/1
  Compare To Constant56/1 -> Switch20/2
  Compare To Constant55/1 -> Switch19/2
  mstate/1 -> Compare To Constant/1, Compare To Constant2/1, Compare To Constant4/1, Compare To Constant8/1, Compare To Constant10/1, Compare To Constant15/1, Compare To Constant18/1, Compare To Constant21/1, Compare To Constant24/1, Compare To Constant30/1, Compare To Constant34/1, Compare To Constant38/1, Compare To Constant42/1, Compare To Constant46/1, Compare To Constant50/1, Compare To Constant54/1, Compare To Constant55/1, Compare To Constant27/1, Compare To Constant12/1, Compare To Constant6/1
  Switch19/1 -> Switch18/3
  Compare To Constant54/1 -> Switch18/2
  Switch18/1 -> Switch17/3
  not15/1 -> and17/6
  Switch17/1 -> Switch16/3
  Compare To Constant52/1 -> and17/3
  mission1_status/1 -> Switch2/1, Switch3/1, Switch6/1, Switch7/1, Switch8/1, Switch9/1, Switch10/1, Switch11/1, Switch12/1, Switch13/1, Switch14/1, Switch15/1, Switch16/1, Switch17/1, Switch18/1, Switch21/1, Switch22/1, Switch22/3, Compare To Constant1/1, Compare To Constant3/1, Compare To Constant5/1, Compare To Constant9/1, Compare To Constant11/1, Compare To Constant13/1, Compare To Constant16/1, Compare To Constant19/1, Compare To Constant22/1, Compare To Constant25/1, Compare To Constant28/1, Compare To Constant31/1, Compare To Constant35/1, Compare To Constant39/1, Compare To Constant43/1, Compare To Constant47/1, Compare To Constant51/1, Compare To Constant56/1, Compare To Constant7/1
  Compare To Constant50/1 -> and17/1
  Compare To Constant53/1 -> and17/5
  dest_reached/1 -> not3/1, and3/3, and4/3, and5/3, not6/1, and7/4, not8/1, and10/4, and11/4, not11/1, and13/4, not13/1, and15/4, and17/4, and16/4, and9/4, not1/1, and2/3
  mission2_status/1 -> Compare To Constant20/1, Compare To Constant23/1, Compare To Constant26/1, Compare To Constant29/1, Compare To Constant32/1, Compare To Constant36/1, Compare To Constant40/1, Compare To Constant44/1, Compare To Constant48/1, Compare To Constant52/1, Compare To Constant57/1, Compare To Constant17/1, Compare To Constant14/1
  Compare To Constant51/1 -> and17/2
  and17/1 -> Switch17/2
  Compare To Constant49/1 -> and16/5
  Compare To Constant47/1 -> and16/2
  Compare To Constant48/1 -> and16/3
  and16/1 -> Switch16/2
  Compare To Constant46/1 -> and16/1
  Switch16/1 -> Switch15/3
  Compare To Constant43/1 -> and15/2
  Compare To Constant42/1 -> and15/1
  not14/1 -> and15/6
  Switch15/1 -> Switch14/3
  Compare To Constant44/1 -> and15/3
  Compare To Constant45/1 -> and15/5
  and15/1 -> Switch15/2
  not13/1 -> and14/4
  and14/1 -> Switch14/2
  Switch14/1 -> Switch13/3
  Compare To Constant41/1 -> and14/5
  Compare To Constant38/1 -> and14/1
  Compare To Constant39/1 -> and14/2
  Compare To Constant40/1 -> and14/3
  not12/1 -> and13/6
  Compare To Constant36/1 -> and13/3
  Compare To Constant35/1 -> and13/2
  Compare To Constant34/1 -> and13/1
  and13/1 -> Switch13/2
  Compare To Constant37/1 -> and13/5
  Switch13/1 -> Switch12/3
  Compare To Constant33/1 -> and12/5
  not11/1 -> and12/4
  Compare To Constant32/1 -> and12/3
  and12/1 -> Switch12/2
  Compare To Constant31/1 -> and12/2
  Switch12/1 -> Switch11/3
  Compare To Constant30/1 -> and12/1
  not10/1 -> and11/5
  Compare To Constant27/1 -> and11/1
  Compare To Constant28/1 -> and11/2
  and11/1 -> Switch11/2
  Compare To Constant29/1 -> and11/3
  Switch11/1 -> Switch10/3
  Compare To Constant25/1 -> and10/2
  Compare To Constant26/1 -> and10/3
  Compare To Constant24/1 -> and10/1
  and10/1 -> Switch10/2
  Switch10/1 -> Switch9/3
  not9/1 -> and9/5
  Compare To Constant22/1 -> and9/2
  and9/1 -> Switch9/2
  Compare To Constant23/1 -> and9/3
  Compare To Constant21/1 -> and9/1
  Switch9/1 -> Switch8/3
  not8/1 -> and8/4
  Compare To Constant19/1 -> and8/2
  Switch8/1 -> Switch7/3
  and8/1 -> Switch8/2
  Compare To Constant20/1 -> and8/3
  Compare To Constant18/1 -> and8/1
  not7/1 -> and7/5
  Switch7/1 -> Switch6/3
  Compare To Constant15/1 -> and7/1
  Compare To Constant16/1 -> and7/2
  and7/1 -> Switch7/2
  Compare To Constant17/1 -> and7/3
  Compare To Constant14/1 -> and6/3
  and6/1 -> Switch6/2
  Switch6/1 -> Switch5/3
  not6/1 -> and6/4
  Compare To Constant12/1 -> and6/1
  Compare To Constant13/1 -> and6/2
  Switch5/1 -> Switch4/3
  not5/1 -> and5/4
  and5/1 -> Switch5/2
  Compare To Constant11/1 -> and5/2
  Compare To Constant10/1 -> and5/1
  Switch4/1 -> Switch3/3
  Compare To Constant9/1 -> and4/2
  and4/1 -> Switch4/2
  Compare To Constant8/1 -> and4/1
  not4/1 -> and3/4
  Compare To Constant6/1 -> and3/1
  Switch3/1 -> Switch2/3
  Compare To Constant7/1 -> and3/2
  and3/1 -> Switch3/2
  not3/1 -> and1/3
  and1/1 -> Switch2/2
  Compare To Constant5/1 -> and1/2
  Compare To Constant4/1 -> and1/1
  Switch2/1 -> Switch1/3
  not2/1 -> and2/4
  and2/1 -> Switch1/2
  Switch1/1 -> Switch/3
  Compare To Constant2/1 -> and2/1
  Compare To Constant3/1 -> and2/2
  not1/1 -> and101/3
  Compare To Constant1/1 -> and101/2
  Compare To Constant/1 -> and101/1
  and101/1 -> Switch/2
  Switch/1 -> upd_mission1_status/1
  Constant/1 -> Switch/1
  Constant1/1 -> Switch1/1
  Constant2/1 -> Switch4/1
  Constant3/1 -> Switch5/1
  c11/1 -> Switch19/3
